simulink model "one_subtractor"  (R2018a)
settings: Solver=VariableStepAuto  StartTime=0.0  StopTime=10.0  RelTol=1e-3
settings Model: Creator=Edoardo Debenedetti  LastModifiedBy=Edoardo Debenedetti

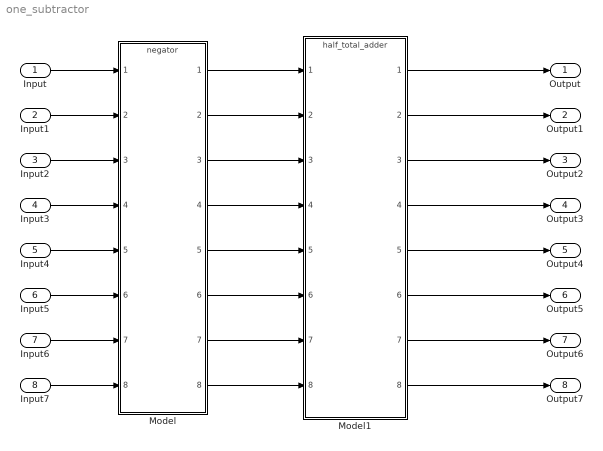
== system one_subtractor ==
  Input : Inport
  Input1 : Inport  Port=2
  Input2 : Inport  Port=3
  Input3 : Inport  Port=4
  Input4 : Inport  Port=5
  Input5 : Inport  Port=6
  Input6 : Inport  Port=7
  Input7 : Inport  Port=8
  Model : ModelReference  ModelNameDialog=negator  SimulationMode=Normal  ModelReferenceVersion=1.2
  Model1 : ModelReference  ModelNameDialog=half_total_adder  SimulationMode=Normal  ModelReferenceVersion=1.2
  Output : Outport
  Output1 : Outport  Port=2
  Output2 : Outport  Port=3
  Output3 : Outport  Port=4
  Output4 : Outport  Port=5
  Output5 : Outport  Port=6
  Output6 : Outport  Port=7
  Output7 : Outport  Port=8
  wires:
  Input/1 -> Model/1
  Input1/1 -> Model/2
  Input3/1 -> Model/4
  Input2/1 -> Model/3
  Input6/1 -> Model/7
  Input7/1 -> Model/8
  Input5/1 -> Model/6
  Input4/1 -> Model/5
  Model/1 -> Model1/1
  Model/2 -> Model1/2
  Model/3 -> Model1/3
  Model/4 -> Model1/4
  Model/5 -> Model1/5
  Model/6 -> Model1/6
  Model/7 -> Model1/7
  Model/8 -> Model1/8
  Model1/1 -> Output/1
  Model1/2 -> Output1/1
  Model1/4 -> Output3/1
  Model1/3 -> Output2/1
  Model1/7 -> Output6/1
  Model1/8 -> Output7/1
  Model1/6 -> Output5/1
  Model1/5 -> Output4/1
